simulink model "sf_slalgo"  (R2017b)
settings: Solver=FixedStepDiscrete  StartTime=0.0  StopTime=10.0  FixedStep=.01  RelTol=1e-3  EnableMultiTasking=on
settings Model: Creator=The MathWorks, Inc.  LastModifiedBy=The MathWorks, Inc.
settings DataIOCC: LimitDataPoints=on  SaveFormat=Array
settings OptimizationCC: ExpressionDepthLimit=2147483647  LifeSpan=inf
settings DebuggingCC: UnderspecifiedInitializationDetection=Classic  MergeDetectMultiDrivingBlocksExec=none  SolverPrmCheckMsg=warning  FcnCallInpInsideContextMsg=warning  StateNameClashWarn=warning  StrictBusMsg=Warning  SFUnexpectedBacktrackingDiag=warning  SFNoUnconditionalDefaultTransitionDiag=warning  SFExecutionAtInitializationDiag=none
settings HardwareCC: ProdBitPerPointer=32  ProdBitPerSizeT=32  ProdBitPerPtrDiffT=32  ProdLargestAtomicFloat=None  ProdIntDivRoundTo=Undefined  ProdEndianess=Unspecified  ProdWordSize=32  ProdHWDeviceType=32-bit Generic
settings ModelReferenceCC: PropagateSignalLabelsOutOfModel=off
settings SFSimCC: SimParseCustomCode=off
settings CodeAppCC: StateflowObjectComments=on
settings GRTTargetCC: TargetLangStandard=C89/C90 (ANSI)  GeneratePreprocessorConditionals=Disable all  CombineOutputUpdateFcns=off  GRTInterface=on
settings ConfigComp: CovMetricSettings=dw  CovHtmlReporting=on  CovSaveCumulativeToWorkspaceVar=on  CovSaveSingleToWorkspaceVar=on  CovExternalEMLEnable=off  CovSFcnEnable=off

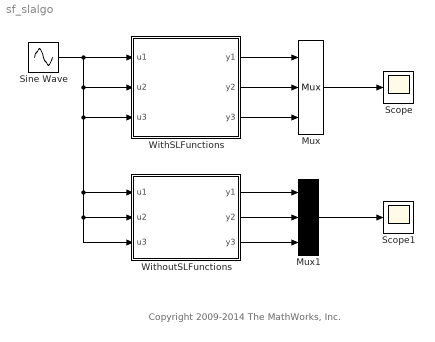
== system sf_slalgo ==
  note: Copyright 2009-2014 The MathWorks, Inc.
  Mux : Mux  Inputs=3
  Mux1 : Mux  Inputs=3
  Scope : Scope
  Scope1 : Scope
  Sine Wave : Sin  SampleTime=0
  WithSLFunctions : Stateflow chart  TreatAsAtomicUnit=on
  WithoutSLFunctions : Subsystem
  wires:
  Sine Wave/1 -> WithSLFunctions/1(u1), WithSLFunctions/2(u2), WithSLFunctions/3(u3), WithoutSLFunctions/1(u1), WithoutSLFunctions/2(u2), WithoutSLFunctions/3(u3)
  WithSLFunctions/1(y1) -> Mux/1
  WithSLFunctions/2(y2) -> Mux/2
  WithSLFunctions/3(y3) -> Mux/3
  Mux/1 -> Scope/1
  WithoutSLFunctions/1(y1) -> Mux1/1
  WithoutSLFunctions/2(y2) -> Mux1/2
  WithoutSLFunctions/3(y3) -> Mux1/3
  Mux1/1 -> Scope1/1

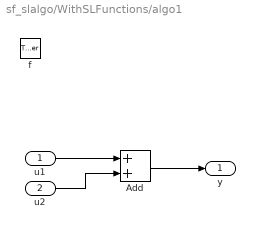
== system sf_slalgo/WithSLFunctions/algo1 ==
  u1 : Inport
  u2 : Inport  Port=2
  f : TriggerPort  TriggerType=function-call  VariantControl=(inherit)
      settings: CopyFcn=Stateflow.SLINSF.SimulinkMan.removeBlockPreDeleteFcn  PreDeleteFcn=Stateflow.SLINSF.SimulinkMan.unsafePredeleteFcn
  Add : Sum
  y : Outport
  wires:
  Add/1 -> y/1
  u2/1 -> Add/2
  u1/1 -> Add/1

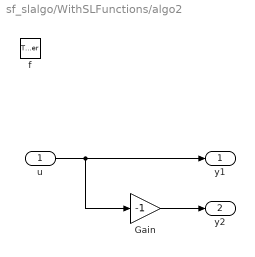
== system sf_slalgo/WithSLFunctions/algo2 ==
  u : Inport
  f : TriggerPort  TriggerType=function-call  VariantControl=(inherit)
      settings: CopyFcn=Stateflow.SLINSF.SimulinkMan.removeBlockPreDeleteFcn  PreDeleteFcn=Stateflow.SLINSF.SimulinkMan.unsafePredeleteFcn
  Gain : Gain  Gain=-1
  y1 : Outport
  y2 : Outport  Port=2
  wires:
  Gain/1 -> y2/1
  u/1 -> Gain/1, y1/1

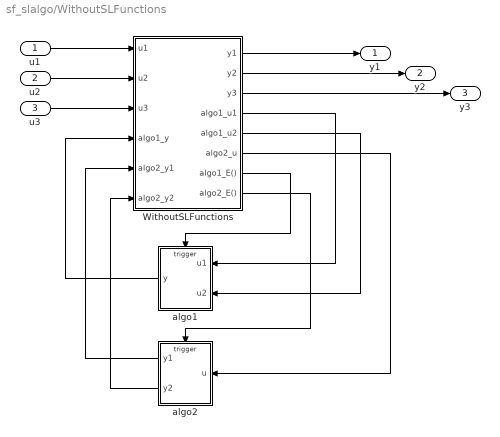
== system sf_slalgo/WithoutSLFunctions ==
  u1 : Inport
  u2 : Inport  Port=2
  u3 : Inport  Port=3
  WithoutSLFunctions : Stateflow chart  TreatAsAtomicUnit=on
  algo1 : Subsystem
      settings: UndoDeleteFcn=sfprivate('simfcn_man','restorePreDeleteFcn')  PreDeleteFcn=sfprivate('simfcn_man','removePreDeleteFcn')
  algo2 : Subsystem
      settings: UndoDeleteFcn=sfprivate('simfcn_man','restorePreDeleteFcn')  PreDeleteFcn=sfprivate('simfcn_man','removePreDeleteFcn')
  y1 : Outport
  y2 : Outport  Port=2
  y3 : Outport  Port=3
  wires:
  WithoutSLFunctions/1(y1) -> y1/1
  WithoutSLFunctions/2(y2) -> y2/1
  WithoutSLFunctions/3(y3) -> y3/1
  WithoutSLFunctions/4(algo1_u1) -> algo1/1(u1)
  WithoutSLFunctions/5(algo1_u2) -> algo1/2(u2)
  WithoutSLFunctions/6(algo2_u) -> algo2/1(u)
  algo1/1(y) -> WithoutSLFunctions/4(algo1_y)
  algo2/1(y1) -> WithoutSLFunctions/5(algo2_y1)
  algo2/2(y2) -> WithoutSLFunctions/6(algo2_y2)
  WithoutSLFunctions/7(algo1_E()) -> algo1/Trigger
  WithoutSLFunctions/8(algo2_E()) -> algo2/Trigger
  u1/1 -> WithoutSLFunctions/1(u1)
  u2/1 -> WithoutSLFunctions/2(u2)
  u3/1 -> WithoutSLFunctions/3(u3)

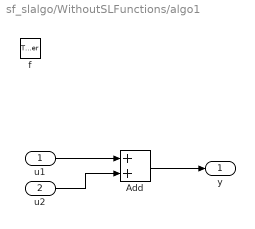
== system sf_slalgo/WithoutSLFunctions/algo1 ==
  u1 : Inport
  u2 : Inport  Port=2
  f : TriggerPort  TriggerType=function-call  VariantControl=(inherit)
      settings: CopyFcn=set_param(gcbh,'PreDeleteFcn','')
  Add : Sum
  y : Outport
  wires:
  u1/1 -> Add/1
  u2/1 -> Add/2
  Add/1 -> y/1

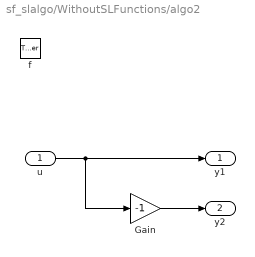
== system sf_slalgo/WithoutSLFunctions/algo2 ==
  u : Inport
  f : TriggerPort  TriggerType=function-call  VariantControl=(inherit)
      settings: CopyFcn=set_param(gcbh,'PreDeleteFcn','')
  Gain : Gain  Gain=-1
  y1 : Outport
  y2 : Outport  Port=2
  wires:
  u/1 -> y1/1, Gain/1
  Gain/1 -> y2/1

== stateflow chart sf_slalgo/WithSLFunctions ==
  state A
    du:
    y1 = algo1(u1,u2)*3;
    [y2,y3] = algo2(u3);
  state y = algo1(u1,u2) [function]
  state [y1,y2] = algo2(u) [function]
  (default) -> A
  data: u1 function_input; u2 function_input; y function_output; u function_input; y1 function_output; y2 function_output; u1 input double; u2 input double; u3 input double; y1 output double; y2 output double; y3 output double

== stateflow chart sf_slalgo/WithoutSLFunctions/WithoutSLFunctions ==
  state A
    du:
    // y1 = algo1(u1,u2)*3
    algo1_u1 = u1;
    algo1_u2 = u2;
    send(algo1_E);
    y1 = algo1_y*3;
    //[y2,y3] = algo2(u3);
    algo2_u = u3;
    send(algo2_E);
    y2 = algo2_y1;
    y3 = algo2_y2;
  (default) -> A
  data: u1 input double; u2 input double; u3 input double; y1 output double; y2 output double; y3 output double; algo1_u1 output double; algo1_u2 output double; algo1_y input double; algo2_u output double; algo2_y1 input double; algo2_y2 input double
  events: algo1_E output FUNCTION_CALL_EVENT; algo2_E output FUNCTION_CALL_EVENT
